simulink model "DAS"  (R2012b)
settings: Solver=FixedStepDiscrete  StartTime=0.0  StopTime=inf  FixedStep=0.1  RelTol=1e-3
PreLoadFcn:
  | if exist('tl_preloadfcn','file'), tl_preloadfcn(gcs,101); end
PostLoadFcn:
  | if exist('tl_postloadfcn','file'), tl_postloadfcn(gcs,101); end
InitFcn:
  | if exist('tlds_init','file'), tlds_init(gcs); end
StartFcn:
  | if exist('tlds_start','file'), tlds_start(gcs); end
StopFcn:
  | if exist('tlds_stop','file'), tlds_stop(gcs); end
undefined symbols (not defined in the file): A, B, C, Dd, DEMO_FAS_Accusti_Threshold_Time, DEMO_FAS_BrakeBooster_Threshold, DEMO_FAS_CC_DELTA, DEMO_FAS_CC_Lvl2_Round, DEMO_FAS_CC_Min_Value, DEMO_FAS_Distance_Treshold_Far, DEMO_FAS_Distance_Treshold_Med, DEMO_FAS_Distance_Treshold_Near, DEMO_FAS_Distronic, DEMO_FAS_Emerg_Brake_Force1, DEMO_FAS_Emerg_Brake_Force2, DEMO_FAS_Emerg_Brake_Time1, DEMO_FAS_Emerg_Brake_Time2, DEMO_FAS_EmergencyBrake, DEMO_FAS_FollowToStop, DEMO_FAS_Limiter, DEMO_FAS_Limiter_DELTA, DEMO_FAS_Neg_Max_ms, DEMO_FAS_Opti_Threshold_Time, DEMO_FAS_Repeater, DEMO_FAS_Repeater_Time, DEMO_FAS_Signdetection, DEMO_FAS_Tempomat
(part 1 of 11)
PreSaveFcn:
  | if exist('tl_presavefcn','file'), tl_presavefcn(gcs); end
settings Model: TL_MAIN_DATA={'date',735360.45236349537}  TLRevision=101  DS_PROJECTFILE=Oeffentlicher_Demonstrator_FAS.dd  BufferReuse=off  Creator=YVEDUHR  LastModifiedBy=alex
settings OptimizationCC: BlockReduction=off  OptimizeBlockIOStorage=off  BufferReuse=off  ExpressionFolding=off  LocalBlockOutputs=off
settings DebuggingCC: InheritedTsInSrcMsg=none

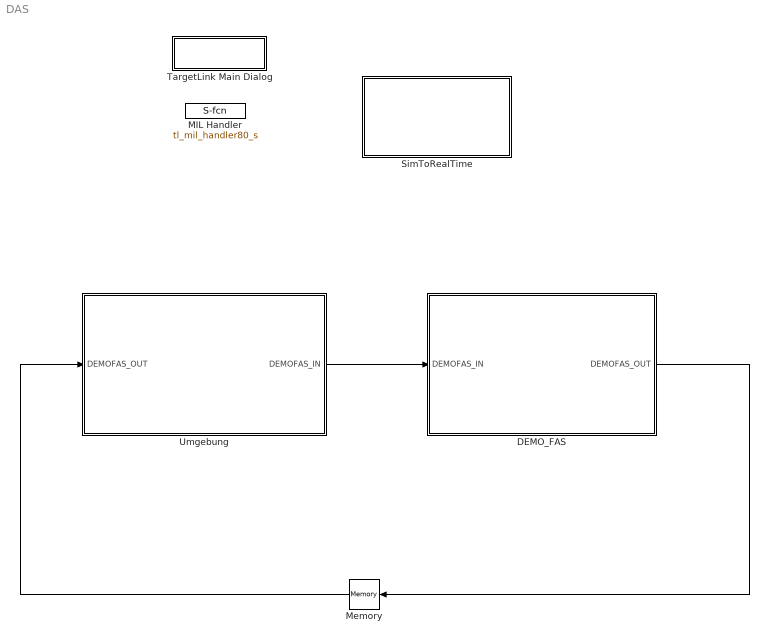
== system DAS ==
  DEMO_FAS : Subsystem
  MIL Handler : S-Function  FunctionName=tl_mil_handler80_s  EnableBusSupport=off  mask(TL_MilHandler){data={'date',730486}}
      mask help: TargetLink MIL Handler
      mask init:
      | fname = sprintf('tl_mil_handler%d_s', 10*get_param(0,'Version'));
      | set_param(gcbh,'FunctionName', fname, 'SFunctionModules','''''');
      settings: DeleteFcn=if exist('delete_tlblock','file')==2,delete_tlblock(gcbh);end  NameChangeFcn=if exist('rename_tlblock','file')==2,rename_tlblock(gcbh);end  OpenFcn=open_system(gcbh,'mask')
      mask Help: eval('if exist(''tl_online_help'',''file'') == 2, tl_online_help(''Topic'',get_param(gcbh,''MaskType'')),end')
      mask Display: disp('MIL Handler')
  Memory : Memory
  SimToRealTime : Subsystem
  TargetLink Main Dialog : Subsystem  mask(TL_MainDialog){data=[]}
      mask help: TargetLink Main Dialog block: In full-featured mode it provides the main graphical user interface to TargetLink.
      mask init:
      | if exist('tl_get_blockset_mode','file')==2
      |    if strcmp(tl_get_blockset_mode,'full-featured')
      |       set_param(gcbh,'BackgroundColor','green');
      |    else
      |       set_param(gcbh,'BackgroundColor','[0.6,0.6,0.6]');
      |    end
      | else
      |    set_param(gcbh,'BackgroundColor','[0.6,0.6,0.6]');
      | end
      settings: CopyFcn=if exist('tl_copyfcn') == 2, tl_copyfcn(gcbh); end
      settings: OpenFcn=|
      | if exist('tl_open_blockdlg','file')==2
      |     tl_open_blockdlg(gcbh);
      | else
      |     open_system(gcbh,'mask');
      | end
      mask Help: eval('if exist(''tl_online_help'',''file'') == 2, tl_online_help(''Topic'',get_param(gcbh,''MaskType'')),end')
      mask Display: disp('TargetLink')
  Umgebung : Subsystem
  wires:
  DEMO_FAS/1(DEMOFAS_OUT) -> Memory/1
  Memory/1 -> Umgebung/1(DEMOFAS_OUT)
  Umgebung/1(DEMOFAS_IN) -> DEMO_FAS/1(DEMOFAS_IN)

== system DAS/DEMO_FAS ==
  DEMOFAS_IN : Inport
  Bus Creator : BusCreator  Inputs=8
  Bus Selector : BusSelector  OutputSignals=ParkingBrake_b,BrakeForce_pedal_pc,Accelaration_pedal_pc,CruiseControl_b,Limiter_b,LeverUp_stat,LeverDown_stat,V_Vehicle_kmh,V_Sign_kmh,Sign_b,Distance_stat,V_Obj_rel_kmh,Distance_Object_m
  DEMO_FAS : Subsystem  Tag=TargetLink Simulation Frame  mask(TL_SimFrame){}
      settings: CopyFcn=if exist('tl_copyfcn','file'), tl_copyfcn(gcbh); end  NameChangeFcn=if exist('tl_framenamechangefcn','file'), tl_framenamechangefcn(gcbh); end
      settings: OpenFcn=|
      | if exist('open_tlsubsystem','file')
      |    open_tlsubsystem(gcbh);
      | else
      |    tlsubsystem = ...
      |       find_system(gcb, ...
      |       'LookUnderMasks','on', ...
      |       'FollowLinks','on', ...
      |       'Tag','MIL Subsystem');
      |    open_system(tlsubsystem);
      | end
      mask Display: disp('TargetLink\nModel-\nin-the-loop\nmode')
  DEMOFAS_OUT : Outport
  wires:
  Bus Creator/1 -> DEMOFAS_OUT/1
  DEMOFAS_IN/1 -> Bus Selector/1
  DEMO_FAS/3(_BrakeForce_pc) -> Bus Creator/3
  DEMO_FAS/6(_Limiter_active_b) -> Bus Creator/6
  DEMO_FAS/5(_LimiterSetValue_kmh) -> Bus Creator/5
  DEMO_FAS/4(_CCSetValue_kmh) -> Bus Creator/4
  DEMO_FAS/2(_Acceleration_pc) -> Bus Creator/2
  DEMO_FAS/1(_CC_active_b) -> Bus Creator/1
  Bus Selector/12 -> DEMO_FAS/12(_V_Obj_rel_kmh)  "<V_Obj_rel_kmh>"
  Bus Selector/13 -> DEMO_FAS/13(_Distance_Object_m)  "<Distance_Object_m>"
  Bus Selector/10 -> DEMO_FAS/10(_Sign_b)  "<Sign_b>"
  Bus Selector/9 -> DEMO_FAS/9(_V_Sign_kmh)  "<V_Sign_kmh>"
  Bus Selector/3 -> DEMO_FAS/3(_Accelaration_pedal_pc)  "<Accelaration_pedal_pc>"
  Bus Selector/4 -> DEMO_FAS/4(_CruiseControl_b)  "<CruiseControl_b>"
  Bus Selector/5 -> DEMO_FAS/5(_Limiter_b)  "<Limiter_b>"
  Bus Selector/2 -> DEMO_FAS/2(_BrakeForce_pedal_pc)  "<BrakeForce_pedal_pc>"
  Bus Selector/7 -> DEMO_FAS/7(_LeverDown_stat)  "<LeverDown_stat>"
  Bus Selector/6 -> DEMO_FAS/6(_LeverUp_stat)  "<LeverUp_stat>"
  Bus Selector/1 -> DEMO_FAS/1(_ParkingBrake_b)  "<ParkingBrake_b>"
  Bus Selector/8 -> DEMO_FAS/8(_V_Vehicle_kmh)  "<V_Vehicle_kmh>"
  Bus Selector/11 -> DEMO_FAS/11(_Distance_stat)  "<Distance_stat>"
  DEMO_FAS/7(_Opti_warn_b) -> Bus Creator/7
  DEMO_FAS/8(_Acusti_warn_b) -> Bus Creator/8

== system DAS/SimToRealTime ==
  Constant : Constant  Value=0
  Constant1 : Constant
  Terminator{,1..5} (6 alike) : Terminator
  VAPS_TimeConfiguration : Subsystem  mask(SL_ACT_SG_VAPS_TimeConfiguration_V100){ts=-1}
      mask prompts: ts "Sample Time"
      mask help:
      | This Blocks syncs if possible the simulation with the real time clock
      | with special features for VAPS
      |
      | This Block has the following Inputs- and Output Signals
      |
      | Input:
      | - TimeConfig: Value [from -10 to 10] to increase or decrease the simulation speed
      |
      | Example:
      |
      | Value:            -10 | -9 | -8 | -7 | -6 | -5 | -4 | -3 | -2 | -1| 0 | 1 | 2 | 3 | 4 | 5 | 6 | 7 | 8 | 9 | 10
      | -----------------------------------------------------------------------------------------------------------------------------------
      | TimeFactor:    0.1|0.9|0.8|0.7|0.6|0.5|0.4|0.3|0.2|0.1| 1 | 1 | 2 | 3 | 4 | 5 | 6 | 7 | 8 | 9 | 10
      |
      | TimeConfig=10 --> :Run 10x faster than Real Time
      | TimeConfig= -5 --> :Run 0.5x as fast than Real Time
      |
      |   -  -1< TimeConfig < 1  	: Run at Real Time
      |    - TimeConfig >1	: Run faster than RealTime
      |    - TimeConfig <-1	: Run slower than RealTime
      |
      | - MaxSpeed:
      |    - MaxSpeed =1	: Run at Real Time with TimeFactor
      |    - MaxSpeed =2	: Run as fast as possible
      |
      | Output:
      | - Factor_SimTime: TimeFactor for the execution SampleTime
      | - TimeConfig_Consumer: TimeConfig for VAPS TimeFactor_Consumer
      | - TimeConfig_Producer: TimeConfig for writing into the TimeConfig_Producer channel
      | - TsSim: SampleTime of the Simulation
      | - TsRTime:Realtime execution SampleTime
      | - TsRTimeEffective: Effective Realtime execution Time
      |
      | Parameter:
      | - Sample Time: execution SampleTime
  wires:
  Constant/1 -> VAPS_TimeConfiguration/1(TimeConfig)
  Constant1/1 -> VAPS_TimeConfiguration/2(MaxSpeed)
  VAPS_TimeConfiguration/1(Factor_SimTime) -> Terminator/1
  VAPS_TimeConfiguration/2(TimeConfig_Consumer) -> Terminator1/1
  VAPS_TimeConfiguration/6(TsRTimeEff) -> Terminator5/1
  VAPS_TimeConfiguration/5(TsRTime) -> Terminator4/1
  VAPS_TimeConfiguration/4(TsSim) -> Terminator3/1
  VAPS_TimeConfiguration/3(TimeConfig_Producer) -> Terminator2/1

== system DAS/TargetLink Main Dialog ==
  dSPACE logo : Subsystem
      mask Display: image(ds_get_icon('dspace_logo_bg_white_l'))

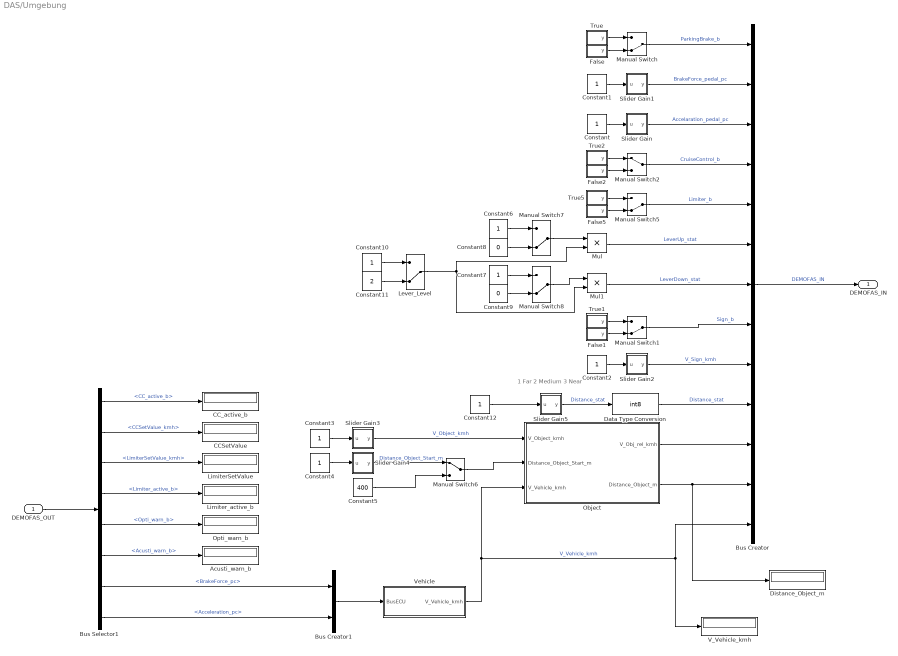
== system DAS/Umgebung ==
  note: 1 Far
      | 2 Medium
      | 3 Near
  DEMOFAS_OUT : Inport
  Acusti_warn_b : Display
  Bus Selector1 : BusSelector  OutputSignals=CC_active_b,CCSetValue_kmh,LimiterSetValue_kmh,Limiter_active_b,Opti_warn_b,Acusti_warn_b,BrakeForce_pc,Acceleration_pc
  Bus Creator : BusCreator  Inputs=13
  Bus Creator1 : BusCreator  Inputs=2
  CCSetValue : Display
  CC_active_b : Display
  Constant{,1..4,6..7,10,12} (9 alike) : Constant
  Constant11 : Constant  Value=2
  Constant5 : Constant  Value=400
  Constant8 : Constant  Value=0
  Constant9 : Constant  Value=0
  Data Type Conversion : DataTypeConversion  OutMin=1  OutMax=3  OutDataTypeStr=int8
  Distance_Object_m : Display
  False : Subsystem  mask(ACT_SG_V200_False){}
      mask help: False
      mask Display: disp('False');
  False1 : Subsystem  mask(ACT_SG_V200_False){}
      mask help: False
      mask Display: disp('False');
  False2 : Subsystem  mask(ACT_SG_V200_False){}
      mask help: False
      mask Display: disp('False');
  False5 : Subsystem  mask(ACT_SG_V200_False){}
      mask help: False
      mask Display: disp('False');
  Lever_Level : ManualSwitch  CurrentSetting=0
  LimiterSetValue : Display
  Limiter_active_b : Display
  Manual Switch{,1,5,7..8} (5 alike) : ManualSwitch  CurrentSetting=0
  Manual Switch2 : ManualSwitch
  Manual Switch6 : ManualSwitch
  Mul : Product  SaturateOnIntegerOverflow=on  InputSameDT=on  OutDataTypeStr=Inherit: Same as first input
  Mul1 : Product  SaturateOnIntegerOverflow=on  InputSameDT=on  OutDataTypeStr=Inherit: Same as first input
  Object : Subsystem
  Opti_warn_b : Display
  Slider Gain : Subsystem  LoadFcn=slideg Load  StartFcn=slideg StartFcn  StopFcn=slideg StopFcn  mask(Slider Gain){low=0, gain=50, high=100}
      mask prompts: low "Simulink:masks:Low_MP"; gain "Simulink:masks:Gain_MP"; high "Simulink:masks:High_MP"
      settings: CopyFcn=slideg Copy  DeleteFcn=slideg DeleteBlock  NameChangeFcn=slideg NameChange  OpenFcn=slideg Open  CloseFcn=slideg Close  ParentCloseFcn=slideg ParentClose
      mask Display: disp(gain)
  Slider Gain1 : Subsystem  LoadFcn=slideg Load  StartFcn=slideg StartFcn  StopFcn=slideg StopFcn  mask(Slider Gain){low=0, gain=0, high=100}
      mask prompts: low "Simulink:masks:Low_MP"; gain "Simulink:masks:Gain_MP"; high "Simulink:masks:High_MP"
      settings: CopyFcn=slideg Copy  DeleteFcn=slideg DeleteBlock  NameChangeFcn=slideg NameChange  OpenFcn=slideg Open  CloseFcn=slideg Close  ParentCloseFcn=slideg ParentClose
      mask Display: disp(gain)
  Slider Gain2 : Subsystem  LoadFcn=slideg Load  StartFcn=slideg StartFcn  StopFcn=slideg StopFcn  mask(Slider Gain){low=0, gain=50, high=100}
      mask prompts: low "Simulink:masks:Low_MP"; gain "Simulink:masks:Gain_MP"; high "Simulink:masks:High_MP"
      settings: CopyFcn=slideg Copy  DeleteFcn=slideg DeleteBlock  NameChangeFcn=slideg NameChange  OpenFcn=slideg Open  CloseFcn=slideg Close  ParentCloseFcn=slideg ParentClose
      mask Display: disp(gain)
  Slider Gain3 : Subsystem  LoadFcn=slideg Load  StartFcn=slideg StartFcn  StopFcn=slideg StopFcn  mask(Slider Gain){low=0, gain=30, high=250}
      mask prompts: low "Simulink:masks:Low_MP"; gain "Simulink:masks:Gain_MP"; high "Simulink:masks:High_MP"
      settings: CopyFcn=slideg Copy  DeleteFcn=slideg DeleteBlock  NameChangeFcn=slideg NameChange  OpenFcn=slideg Open  CloseFcn=slideg Close  ParentCloseFcn=slideg ParentClose
      mask Display: disp(gain)
  Slider Gain4 : Subsystem  LoadFcn=slideg Load  StartFcn=slideg StartFcn  StopFcn=slideg StopFcn  mask(Slider Gain){low=0, gain=50, high=300}
      mask prompts: low "Simulink:masks:Low_MP"; gain "Simulink:masks:Gain_MP"; high "Simulink:masks:High_MP"
      settings: CopyFcn=slideg Copy  DeleteFcn=slideg DeleteBlock  NameChangeFcn=slideg NameChange  OpenFcn=slideg Open  CloseFcn=slideg Close  ParentCloseFcn=slideg ParentClose
      mask Display: disp(gain)
  Slider Gain5 : Subsystem  LoadFcn=slideg Load  StartFcn=slideg StartFcn  StopFcn=slideg StopFcn  mask(Slider Gain){low=1, gain=2.36, high=3}
      mask prompts: low "Simulink:masks:Low_MP"; gain "Simulink:masks:Gain_MP"; high "Simulink:masks:High_MP"
      settings: CopyFcn=slideg Copy  DeleteFcn=slideg DeleteBlock  NameChangeFcn=slideg NameChange  OpenFcn=slideg Open  CloseFcn=slideg Close  ParentCloseFcn=slideg ParentClose
      mask Display: disp(gain)
  True : Subsystem  mask(ACT_SG_V200_True){}
      mask help: True
      mask Display: disp('True')
  True1 : Subsystem  mask(ACT_SG_V200_True){}
      mask help: True
      mask Display: disp('True')
  True2 : Subsystem  mask(ACT_SG_V200_True){}
      mask help: True
      mask Display: disp('True')
  True5 : Subsystem  mask(ACT_SG_V200_True){}
      mask help: True
      mask Display: disp('True')
  V_Vehicle_kmh : Display
  Vehicle : Subsystem
  DEMOFAS_IN : Outport
  wires:
  Bus Creator/1 -> DEMOFAS_IN/1  "DEMOFAS_IN"
  True/1(y) -> Manual Switch/1
  False/1(y) -> Manual Switch/2
  Manual Switch/1 -> Bus Creator/1  "ParkingBrake_b"
  Slider Gain1/1(y) -> Bus Creator/2  "BrakeForce_pedal_pc"
  True2/1(y) -> Manual Switch2/1
  False2/1(y) -> Manual Switch2/2
  Manual Switch2/1 -> Bus Creator/4  "CruiseControl_b"
  True5/1(y) -> Manual Switch5/1
  False5/1(y) -> Manual Switch5/2
  Manual Switch5/1 -> Bus Creator/5  "Limiter_b"
  Vehicle/1(V_Vehicle_kmh) -> Object/3(V_Vehicle_kmh), Bus Creator/13, V_Vehicle_kmh/1  "V_Vehicle_kmh"
  Bus Creator1/1 -> Vehicle/1(BusECU)
  DEMOFAS_OUT/1 -> Bus Selector1/1
  Bus Selector1/8 -> Bus Creator1/2  "<Acceleration_pc>"
  Constant/1 -> Slider Gain/1(u)
  Slider Gain/1(y) -> Bus Creator/3  "Accelaration_pedal_pc"
  Constant1/1 -> Slider Gain1/1(u)
  Bus Selector1/1 -> CC_active_b/1  "<CC_active_b>"
  Bus Selector1/2 -> CCSetValue/1  "<CCSetValue_kmh>"
  Bus Selector1/3 -> LimiterSetValue/1  "<LimiterSetValue_kmh>"
  Bus Selector1/4 -> Limiter_active_b/1  "<Limiter_active_b>"
  Bus Selector1/7 -> Bus Creator1/1  "<BrakeForce_pc>"
  True1/1(y) -> Manual Switch1/1
  False1/1(y) -> Manual Switch1/2
  Manual Switch1/1 -> Bus Creator/8  "Sign_b"
  Constant2/1 -> Slider Gain2/1(u)
  Slider Gain2/1(y) -> Bus Creator/9  "V_Sign_kmh"
  Constant3/1 -> Slider Gain3/1(u)
  Slider Gain3/1(y) -> Object/1(V_Object_kmh)  "V_Object_kmh"
  Constant4/1 -> Slider Gain4/1(u)
  Slider Gain4/1(y) -> Manual Switch6/1  "Distance_Object_Start_m"
  Constant5/1 -> Manual Switch6/2
  Manual Switch6/1 -> Object/2(Distance_Object_Start_m)
  Object/1(V_Obj_rel_kmh) -> Bus Creator/11
  Object/2(Distance_Object_m) -> Distance_Object_m/1, Bus Creator/12
  Constant6/1 -> Manual Switch7/1
  Constant7/1 -> Manual Switch8/1
  Constant8/1 -> Manual Switch7/2
  Constant9/1 -> Manual Switch8/2
  Mul/1 -> Bus Creator/6  "LeverUp_stat"
  Manual Switch7/1 -> Mul/1
  Constant10/1 -> Lever_Level/1
  Constant11/1 -> Lever_Level/2
  Lever_Level/1 -> Mul/2, Mul1/2
  Mul1/1 -> Bus Creator/7  "LeverDown_stat"
  Manual Switch8/1 -> Mul1/1
  Slider Gain5/1(y) -> Data Type Conversion/1  "Distance_stat"
  Constant12/1 -> Slider Gain5/1(u)
  Data Type Conversion/1 -> Bus Creator/10  "Distance_stat"
  Bus Selector1/5 -> Opti_warn_b/1  "<Opti_warn_b>"
  Bus Selector1/6 -> Acusti_warn_b/1  "<Acusti_warn_b>"

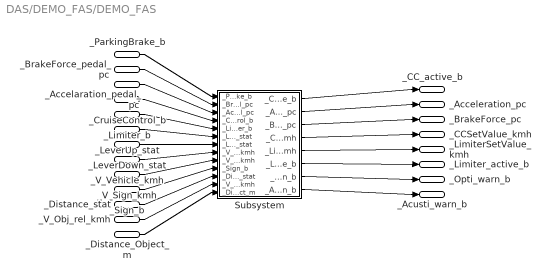
== system DAS/DEMO_FAS/DEMO_FAS ==
  _ParkingBrake_b : Inport
  _BrakeForce_pedal_pc : Inport  Port=2
  _Accelaration_pedal_pc : Inport  Port=3
  _CruiseControl_b : Inport  Port=4
  _Limiter_b : Inport  Port=5
  _LeverUp_stat : Inport  Port=6
  _LeverDown_stat : Inport  Port=7
  _V_Vehicle_kmh : Inport  Port=8
  _V_Sign_kmh : Inport  Port=9
  _Sign_b : Inport  Port=10
  _Distance_stat : Inport  Port=11
  _V_Obj_rel_kmh : Inport  Port=12
  _Distance_Object_m : Inport  Port=13
  Subsystem : Subsystem  Tag=struct('sfcnName','DEMO_FAS_sf','subFunction','','srcSubsystem','')  mask(TL_Enable){}
      settings: OpenFcn=warndlg(get_param(gcb,'MaskHelp'),'Serious Warning');
      mask Help: This subsystem keeps the TargetLink subsystem (subsystem with TargetLink blocks for production code generation), and is needed for the TargetLink simulation frame to work properly. DO NOT DELETE OR MODIFY IT!
  _CC_active_b : Outport
  _Acceleration_pc : Outport  Port=2
  _BrakeForce_pc : Outport  Port=3
  _CCSetValue_kmh : Outport  Port=4
  _LimiterSetValue_kmh : Outport  Port=5
  _Limiter_active_b : Outport  Port=6
  _Opti_warn_b : Outport  Port=7
  _Acusti_warn_b : Outport  Port=8
  wires:
  _ParkingBrake_b/1 -> Subsystem/1(_ParkingBrake_b)
  _BrakeForce_pedal_pc/1 -> Subsystem/2(_BrakeForce_pedal_pc)
  _Accelaration_pedal_pc/1 -> Subsystem/3(_Accelaration_pedal_pc)
  _CruiseControl_b/1 -> Subsystem/4(_CruiseControl_b)
  _Limiter_b/1 -> Subsystem/5(_Limiter_b)
  _LeverUp_stat/1 -> Subsystem/6(_LeverUp_stat)
  _LeverDown_stat/1 -> Subsystem/7(_LeverDown_stat)
  _V_Vehicle_kmh/1 -> Subsystem/8(_V_Vehicle_kmh)
  _V_Sign_kmh/1 -> Subsystem/9(_V_Sign_kmh)
  _Sign_b/1 -> Subsystem/10(_Sign_b)
  _Distance_stat/1 -> Subsystem/11(_Distance_stat)
  _V_Obj_rel_kmh/1 -> Subsystem/12(_V_Obj_rel_kmh)
  _Distance_Object_m/1 -> Subsystem/13(_Distance_Object_m)
  Subsystem/1(_CC_active_b) -> _CC_active_b/1
  Subsystem/2(_Acceleration_pc) -> _Acceleration_pc/1
  Subsystem/3(_BrakeForce_pc) -> _BrakeForce_pc/1
  Subsystem/4(_CCSetValue_kmh) -> _CCSetValue_kmh/1
  Subsystem/5(_LimiterSetValue_kmh) -> _LimiterSetValue_kmh/1
  Subsystem/6(_Limiter_active_b) -> _Limiter_active_b/1
  Subsystem/7(_Opti_warn_b) -> _Opti_warn_b/1
  Subsystem/8(_Acusti_warn_b) -> _Acusti_warn_b/1

== system DAS/SimToRealTime/VAPS_TimeConfiguration ==
  TimeConfig : Inport
  MaxSpeed : Inport  Port=2
  Constant1 : Constant  Value=0
  Constant10 : Constant  Value=2
  Constant4 : Constant  Value=0
  RealTimeTimerAdapter : Subsystem
  RealTimeTimerAdapter_Value : Subsystem
  RelOp4 : RelationalOperator  Operator===  InputSameDT=on
  Switch1 : Switch  Threshold=1  SaturateOnIntegerOverflow=on  InputSameDT=on
  Switch2 : Switch  Threshold=1  SaturateOnIntegerOverflow=on  InputSameDT=on
  SysInit1 : Subsystem  mask(ACT_SG_V200_SysInit){dT=ts, YName=}
      mask prompts: dT "Sample Time"; YName "Y OutName"
      mask help: An inital pulse is generated for for the first block evaluation.
      mask init:
      | sl_act_sg_init_blk;
      mask Help:
      | <P><B>Function:</B></P>
      | <P>The block provides an initial pulse at the output on the first
      | evaluation of the block.<BR> This function can be used for system startup functions to
      | get defined states in the system.</P>
      | 
      | <P><B>In-/Outputs:</B></P>
      | <P><U>Output</U></P>
      | <P>The output shows TRUE at the first cycle, else it shows FALSE.</P>
      mask Display: disp('SysInit');
  VAPSRealTimeTimer : Subsystem  mask(SL_ACT_SG_VAPSRealTimeTimer_V100){}
      mask help:
      | This Blocks syncs if possible the simulation with the real time clock.
      |
      | This Block has the following Inputs- and Output Signals
      |
      | Input:
      | - TimeFactor: Factor to increase or decrease the simulation speed
      |    - TimeFactor =1  	: Run at Real Time
      |    - TimeFactor >1	: Run TimeFactor faster than RealTime
      |    - TimeFactor <1	: Run TimeFactor slower than RealTime
      |    - TimeFactor =0	: Run as fast as possible
      |
      | Output:
      | - TsSim: SampleTime of the Simulation
      | - TsRTime:Realtime execution SampleTime
      | - TsRTimeEffective: Effective Realtime execution Time
  Factor_SimTime : Outport
  TimeConfig_Consumer : Outport  Port=2
  TimeConfig_Producer : Outport  Port=3
  TsSim : Outport  Port=4
  TsRTime : Outport  Port=5
  TsRTimeEff : Outport  Port=6
  wires:
  Switch2/1 -> RealTimeTimerAdapter/1(In1), RealTimeTimerAdapter_Value/1(In1)
  Constant4/1 -> Switch2/1
  SysInit1/1(y) -> Switch2/2
  TimeConfig/1 -> Switch2/3
  RealTimeTimerAdapter/1(Out1) -> Factor_SimTime/1, Switch1/3
  RealTimeTimerAdapter_Value/1(Out1) -> TimeConfig_Consumer/1, TimeConfig_Producer/1
  VAPSRealTimeTimer/1(TsSim) -> TsSim/1
  VAPSRealTimeTimer/2(TsRTime) -> TsRTime/1
  VAPSRealTimeTimer/3(TsRTimeEffective) -> TsRTimeEff/1
  Constant10/1 -> RelOp4/2
  Switch1/1 -> VAPSRealTimeTimer/1(TimeFactor)
  RelOp4/1 -> Switch1/2
  MaxSpeed/1 -> RelOp4/1
  Constant1/1 -> Switch1/1

== system DAS/TargetLink Main Dialog/dSPACE logo ==

== system DAS/Umgebung/False ==
  Zero : Constant  Value=0
  y : Outport
  wires:
  Zero/1 -> y/1

== system DAS/Umgebung/False1 ==
  Zero : Constant  Value=0
  y : Outport
  wires:
  Zero/1 -> y/1

== system DAS/Umgebung/False2 ==
  Zero : Constant  Value=0
  y : Outport
  wires:
  Zero/1 -> y/1

== system DAS/Umgebung/False5 ==
  Zero : Constant  Value=0
  y : Outport
  wires:
  Zero/1 -> y/1

== system DAS/Umgebung/Object ==
  V_Object_kmh : Inport
  Distance_Object_Start_m : Inport  Port=2
  V_Vehicle_kmh : Inport  Port=3
  Accumulator_REL : Subsystem  mask(MSR_V200_AccumulatorResetEnabledLimited){dT=-1, YName=, b_maxName=, b_minName=}
      mask prompts: dT "Sample Time"; YName "Y OutName"; b_maxName "b_max OutName"; b_minName "b_min OutName"
      mask help:
      | 'y' is the sum of all sampled input values 'u', limited to 'MN' and 'MX'.
      | 'E' on FALSE stops the integration.
      | 'R' on TRUE loads initial value 'IV'.
      | 'y' on limit is indicated by 'b_max' and 'b_min' flags.
      mask init:
      | sl_act_sg_init_blk;
      mask Help:
      | <HTML>
      | <HEAD>
      | <META HTTP-EQUIV="Content-Type" CONTENT="text/html; charset=iso-8859-1">
      | <TITLE>Help</TITLE>
      | </HEAD>
      | <BODY>
      | 
      | <B><FONT FACE="Arial"><P>Function:</P>
      | </B><P>The block works as a totalizer of the input signal
      |  <FONT FACE="Courier New">u</FONT>.</P>
      | 
      | <B><P>In-/Outputs:</P>
      | </B>
      | <P><U>Enable</U></P>
      | <P> If the enable input <FONT FACE="Courier New">E</FONT> is '0' the
      | 	 calculation is stopped and the output
      | 	 <FONT FACE="Courier New">y</FONT> shows the last evaluated value.</P>
      | 
      | <P><U>Input</U></P>
      | <P>The block input <FONT FACE="Courier New">u</FONT> must be connected
      | 	 to the input signal.</P>
      | 
      | <U><P>Reset / Initial Value</P>
      | </U><P>If the reset input <FONT FACE="Courier New">R</FONT>
      | <FONT FACE="Arial"> gets a '1' signal the block will output the initial value
      |  <FONT FACE="Courier New">IV</FONT>.</P>
      | 
      | <U><P>Limit Values</P>
      | </U><P>The inputs <FONT FACE="Courier New">MN</FONT> and
      |  <FONT FACE="Courier New">MX</FONT> specify the signal value limits for
      |   <FONT FACE="Courier New">y</FONT>.</P>
      | 
      | <U><P>Output</P>
      | </U><P>The output <FONT FACE="Courier New">y</FONT> shows the totalized
      |  input signal, limited to <FONT FACE="Courier New">MN</FONT> and
      |   <FONT FACE="Courier New">MX</FONT>.<BR>
      | 	 <FONT FACE="Courier New">b_min</FONT>
      | 	 and <FONT FACE="Courier New">b_max</FONT> indicate that the totalized
      | 	  signal has reached the minimum resp. the maximum.</P>
      | </FONT></BODY>
      | </HTML>
      mask Display: image(imread('Accumulator.tif','tif'),[0.25,0.2,0.3,0.6])
  Add : Sum  Inputs=+-
  Constant : Constant  Value=300
  Constant1 : Constant  Value=1000
  Constant2 : Constant  Value=0
  Gain : Gain  Gain=-1/3.6
  Logical Operator : Logic  Operator=NOT  AllPortsSameDT=off  OutDataTypeStr=boolean
  RelOp : RelationalOperator  Operator=>  InputSameDT=on
  Terminator : Terminator
  Terminator1 : Terminator
  V_Obj_rel_kmh : Outport
  Distance_Object_m : Outport  Port=2
  wires:
  V_Object_kmh/1 -> Add/2
  V_Vehicle_kmh/1 -> Add/1
  Add/1 -> Gain/1, V_Obj_rel_kmh/1  "V_Obj_rel_kmh"
  Gain/1 -> Accumulator_REL/3(u)
  Constant/1 -> RelOp/2
  Distance_Object_Start_m/1 -> RelOp/1, Accumulator_REL/6(IV)
  RelOp/1 -> Logical Operator/1, Accumulator_REL/5(R)
  Constant1/1 -> Accumulator_REL/1(MX)
  Constant2/1 -> Accumulator_REL/2(MN)
  Accumulator_REL/1(y) -> Distance_Object_m/1  "Distance_Object_m"
  Logical Operator/1 -> Accumulator_REL/4(E)
  Accumulator_REL/2(b_max) -> Terminator/1
  Accumulator_REL/3(b_min) -> Terminator1/1

== system DAS/Umgebung/Slider Gain ==
  u : Inport
  Slider Gain : Gain  Gain=gain  SaturateOnIntegerOverflow=on  OutDataTypeStr=Inherit: Same as input  ParamDataTypeStr=Inherit: Same as input
  y : Outport
  wires:
  u/1 -> Slider Gain/1
  Slider Gain/1 -> y/1

== system DAS/Umgebung/Slider Gain1 ==
  u : Inport
  Slider Gain : Gain  Gain=gain  SaturateOnIntegerOverflow=on  OutDataTypeStr=Inherit: Same as input  ParamDataTypeStr=Inherit: Same as input
  y : Outport
  wires:
  u/1 -> Slider Gain/1
  Slider Gain/1 -> y/1

== system DAS/Umgebung/Slider Gain2 ==
  u : Inport
  Slider Gain : Gain  Gain=gain  SaturateOnIntegerOverflow=on  OutDataTypeStr=Inherit: Same as input  ParamDataTypeStr=Inherit: Same as input
  y : Outport
  wires:
  u/1 -> Slider Gain/1
  Slider Gain/1 -> y/1

== system DAS/Umgebung/Slider Gain3 ==
  u : Inport
  Slider Gain : Gain  Gain=gain  SaturateOnIntegerOverflow=on  OutDataTypeStr=Inherit: Same as input  ParamDataTypeStr=Inherit: Same as input
  y : Outport
  wires:
  u/1 -> Slider Gain/1
  Slider Gain/1 -> y/1

== system DAS/Umgebung/Slider Gain4 ==
  u : Inport
  Slider Gain : Gain  Gain=gain  SaturateOnIntegerOverflow=on  OutDataTypeStr=Inherit: Same as input  ParamDataTypeStr=Inherit: Same as input
  y : Outport
  wires:
  u/1 -> Slider Gain/1
  Slider Gain/1 -> y/1

== system DAS/Umgebung/Slider Gain5 ==
  u : Inport
  Slider Gain : Gain  Gain=gain  SaturateOnIntegerOverflow=on  OutDataTypeStr=Inherit: Same as input  ParamDataTypeStr=Inherit: Same as input
  y : Outport
  wires:
  u/1 -> Slider Gain/1
  Slider Gain/1 -> y/1

== system DAS/Umgebung/True ==
  One : Constant
  y : Outport
  wires:
  One/1 -> y/1

== system DAS/Umgebung/True1 ==
  One : Constant
  y : Outport
  wires:
  One/1 -> y/1

== system DAS/Umgebung/True2 ==
  One : Constant
  y : Outport
  wires:
  One/1 -> y/1

== system DAS/Umgebung/True5 ==
  One : Constant
  y : Outport
  wires:
  One/1 -> y/1

== system DAS/Umgebung/Vehicle ==
  BusECU : Inport
  Bus Selector : BusSelector  OutputSignals=BrakeForce_pc,Acceleration_pc
  Constant : Constant  Value=0
  Constant1 : Constant  Value=0
  Discrete Transfer Fcn (with initial states) : Subsystem  mask(Discrete Transfer Function with Initial States){N=[0.009975], D=[1  -0.997], X0=[1], TS=.1}
      mask prompts: N "SimulinkBlocks:simulink_extras:Numerator_MP"; D "SimulinkBlocks:simulink_extras:Denominator_MP"; X0 "SimulinkBlocks:simulink_extras:InitialConditions_MP"; TS "SimulinkBlocks:simulink_extras:SampleTime_MP"
      mask help: SimulinkBlocks:simulink_extras:DiscreteTransferFunctionWithInitialStates_MD
      mask init:
      | [A,B,C,Dd]=tf2ss(N,D);if (isempty(X0));[m,n]=size(A);X0=zeros(1,m); end;
      mask Help: Specify the initial states for the transfer function.  The state ordering is determined by the m-file tf2ss.  There is no unique mapping of the states in a transfer function to states in a state-space representation.  However, tf2ss will consistently use the same mapping for a given transfer function.
      mask Display: dpoly(N,D,'z')
  Gain : Gain  Gain=-2
  Relational Operator : RelationalOperator  Operator=<  OutDataTypeStr=boolean
  Saturation : Saturate  UpperLimit=250  LowerLimit=0
  Sum1 : Sum  Inputs=+--  SaturateOnIntegerOverflow=on  InputSameDT=on  OutDataTypeStr=Inherit: Same as first input
  Switch : Switch  Criteria=u2 > Threshold
  Switch1 : Switch  Threshold=1
  Uniform Random Number : UniformRandomNumber  Minimum=0  SampleTime=0.1
  Unit Delay : UnitDelay  SampleTime=-1
  Widerstand : Lookup  InputValues=[0 100 175 250]  Table=[0 8 18 33]  OutMax=[100]
  V_Vehicle_kmh : Outport
  wires:
  Saturation/1 -> Unit Delay/1, V_Vehicle_kmh/1  "V_Vehicle_kmh"
  Gain/1 -> Switch/1
  Switch/1 -> Discrete Transfer Fcn (with initial states)/1(In1)
  BusECU/1 -> Bus Selector/1
  Bus Selector/2 -> Switch/3  "<Acceleration_pc>"
  Sum1/1 -> Saturation/1
  Discrete Transfer Fcn (with initial states)/1(Out1) -> Sum1/1  "V_Vehicle_kmh"
  Widerstand/1 -> Sum1/2
  Unit Delay/1 -> Relational Operator/2, Widerstand/1
  Uniform Random Number/1 -> Sum1/3
  Constant/1 -> Relational Operator/1
  Relational Operator/1 -> Switch1/2
  Bus Selector/1 -> Switch1/1  "<BrakeForce_pc>"
  Switch1/1 -> Switch/2, Gain/1
  Constant1/1 -> Switch1/3

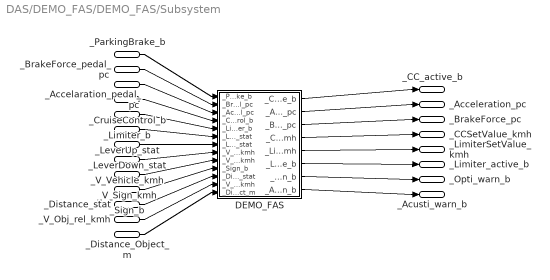
== system DAS/DEMO_FAS/DEMO_FAS/Subsystem ==
  _ParkingBrake_b : Inport
  _BrakeForce_pedal_pc : Inport  Port=2
  _Accelaration_pedal_pc : Inport  Port=3
  _CruiseControl_b : Inport  Port=4
  _Limiter_b : Inport  Port=5
  _LeverUp_stat : Inport  Port=6
  _LeverDown_stat : Inport  Port=7
  _V_Vehicle_kmh : Inport  Port=8
  _V_Sign_kmh : Inport  Port=9
  _Sign_b : Inport  Port=10
  _Distance_stat : Inport  Port=11
  _V_Obj_rel_kmh : Inport  Port=12
  _Distance_Object_m : Inport  Port=13
  DEMO_FAS : Subsystem  Tag=MIL Subsystem  Description=a  mask(MIL Subsystem){}
      settings: CopyFcn=if exist('tl_copyfcn','file'), tl_copyfcn(gcbh); end  NameChangeFcn=if exist('tl_namechangefcn','file'), tl_namechangefcn(gcbh); end  DestroyFcn=if exist('update_tl_main_dlg','file'), update_tl_main_dlg('TL_subs_display'); end
  _CC_active_b : Outport
  _Acceleration_pc : Outport  Port=2
  _BrakeForce_pc : Outport  Port=3
  _CCSetValue_kmh : Outport  Port=4
  _LimiterSetValue_kmh : Outport  Port=5
  _Limiter_active_b : Outport  Port=6
  _Opti_warn_b : Outport  Port=7
  _Acusti_warn_b : Outport  Port=8
  wires:
  _ParkingBrake_b/1 -> DEMO_FAS/1(_ParkingBrake_b)
  _BrakeForce_pedal_pc/1 -> DEMO_FAS/2(_BrakeForce_pedal_pc)
  _Accelaration_pedal_pc/1 -> DEMO_FAS/3(_Accelaration_pedal_pc)
  _CruiseControl_b/1 -> DEMO_FAS/4(_CruiseControl_b)
  _Limiter_b/1 -> DEMO_FAS/5(_Limiter_b)
  _LeverUp_stat/1 -> DEMO_FAS/6(_LeverUp_stat)
  _LeverDown_stat/1 -> DEMO_FAS/7(_LeverDown_stat)
  _V_Vehicle_kmh/1 -> DEMO_FAS/8(_V_Vehicle_kmh)
  _V_Sign_kmh/1 -> DEMO_FAS/9(_V_Sign_kmh)
  _Sign_b/1 -> DEMO_FAS/10(_Sign_b)
  _Distance_stat/1 -> DEMO_FAS/11(_Distance_stat)
  _V_Obj_rel_kmh/1 -> DEMO_FAS/12(_V_Obj_rel_kmh)
  _Distance_Object_m/1 -> DEMO_FAS/13(_Distance_Object_m)
  DEMO_FAS/1(_CC_active_b) -> _CC_active_b/1
  DEMO_FAS/2(_Acceleration_pc) -> _Acceleration_pc/1
  DEMO_FAS/3(_BrakeForce_pc) -> _BrakeForce_pc/1
  DEMO_FAS/4(_CCSetValue_kmh) -> _CCSetValue_kmh/1
  DEMO_FAS/5(_LimiterSetValue_kmh) -> _LimiterSetValue_kmh/1
  DEMO_FAS/6(_Limiter_active_b) -> _Limiter_active_b/1
  DEMO_FAS/7(_Opti_warn_b) -> _Opti_warn_b/1
  DEMO_FAS/8(_Acusti_warn_b) -> _Acusti_warn_b/1

== system DAS/SimToRealTime/VAPS_TimeConfiguration/RealTimeTimerAdapter ==
  In1 : Inport
  Constant1 : Constant  Value=-10
  Constant10 : Constant
  Constant11 : Constant
  Constant12 : Constant  Value=-1
  Constant13 : Constant
  Constant15 : Constant  Value=1.1
  Div1 : Product  Inputs=*/  SaturateOnIntegerOverflow=on  InputSameDT=on  OutDataTypeStr=Inherit: Same as first input
  LogOp1 : Logic
  RelOp2 : RelationalOperator  Operator=>  InputSameDT=on
  RelOp3 : RelationalOperator  Operator=<=  InputSameDT=on
  RelOp4 : RelationalOperator  InputSameDT=on
  Sum : Sum  Inputs=+-  SaturateOnIntegerOverflow=on  InputSameDT=on  OutDataTypeStr=Inherit: Same as first input
  Switch2 : Switch  Threshold=1  SaturateOnIntegerOverflow=on  InputSameDT=on
  Switch3 : Switch  Threshold=1  SaturateOnIntegerOverflow=on  InputSameDT=on
  Out1 : Outport
  wires:
  Div1/1 -> Sum/2
  Constant15/1 -> Sum/1
  Constant1/1 -> Div1/2
  Sum/1 -> Switch3/3
  Constant13/1 -> Switch3/1
  LogOp1/1 -> Switch3/2
  RelOp4/1 -> LogOp1/2
  RelOp3/1 -> LogOp1/1
  Constant12/1 -> RelOp4/2
  Switch3/1 -> Switch2/3
  Constant11/1 -> RelOp3/2
  Switch2/1 -> Out1/1
  RelOp2/1 -> Switch2/2
  Constant10/1 -> RelOp2/2
  In1/1 -> Div1/1, RelOp4/1, RelOp3/1, Switch2/1, RelOp2/1

== system DAS/SimToRealTime/VAPS_TimeConfiguration/RealTimeTimerAdapter_Value ==
  In1 : Inport
  Constant11 : Constant
  Constant12 : Constant  Value=-1
  Constant13 : Constant  Value=0
  LogOp1 : Logic
  RelOp3 : RelationalOperator  Operator=<=  InputSameDT=on
  RelOp4 : RelationalOperator  InputSameDT=on
  Switch3 : Switch  Threshold=1  SaturateOnIntegerOverflow=on  InputSameDT=on
  Out1 : Outport
  wires:
  In1/1 -> RelOp3/1, RelOp4/1, Switch3/3
  Switch3/1 -> Out1/1
  Constant11/1 -> RelOp3/2
  Constant12/1 -> RelOp4/2
  RelOp3/1 -> LogOp1/1
  RelOp4/1 -> LogOp1/2
  LogOp1/1 -> Switch3/2
  Constant13/1 -> Switch3/1

== system DAS/SimToRealTime/VAPS_TimeConfiguration/SysInit1 ==
  Memory_Init : UnitDelay  InitialCondition=1  SampleTime=dT
  Zero_Init : Constant  Value=0  SampleTime=dT
  y : Outport
  wires:
  Zero_Init/1 -> Memory_Init/1
  Memory_Init/1 -> y/1

== system DAS/SimToRealTime/VAPS_TimeConfiguration/VAPSRealTimeTimer ==
  TimeFactor : Inport
  Level-2 M-file S-Function : M-S-Function  FunctionName=VAPSRealTimeTimer
  TsSim : Outport
  TsRTime : Outport  Port=2
  TsRTimeEffective : Outport  Port=3
  wires:
  Level-2 M-file S-Function/3 -> TsRTimeEffective/1  "TsRTimeEffective"
  Level-2 M-file S-Function/2 -> TsRTime/1  "TsRTime"
  Level-2 M-file S-Function/1 -> TsSim/1  "TsSim"
  TimeFactor/1 -> Level-2 M-file S-Function/1

== system DAS/Umgebung/Object/Accumulator_REL ==
  MX : Inport
  MN : Inport  Port=2
  u : Inport  Port=3
  E : Inport  Port=4
  R : Inport  Port=5
  IV : Inport  Port=6
  Limit : Subsystem  mask(MSR_V200_Limit){YName=, b_maxName=, b_minName=}
      mask prompts: YName "Y OutName"; b_maxName "b_max OutName"; b_minName "b_min OutName"
      mask help:
      | Limits the input value 'u' between a maximum 'MX' and a minimum 'MN' value.
      | 'b_max' and 'b_min' indicate that the limit is exceeded.
      mask init:
      | sl_act_sg_init_blk;
      mask Help:
      | <HTML>
      | <HEAD>
      | <META HTTP-EQUIV="Content-Type" CONTENT="text/html; charset=iso-8859-1">
      | <TITLE>Help</TITLE>
      | </HEAD>
      | <BODY>
      | 
      | <B><FONT FACE="Arial"><P>Function:</P>
      | </B><P>The block limits the input signal
      |  <FONT FACE="Courier New">u</FONT> to a maximum value
      |   <FONT FACE="Courier New">MX</FONT> and a minimum value
      | 	 <FONT FACE="Courier New">MN</FONT>. First,
      | 	 <FONT FACE="Courier New">u</FONT> is checked against the maximum value,
      | 		then against the minimum value. The outputs
      | 	  <FONT FACE="Courier New">b_min</FONT> and
      | 		 <FONT FACE="Courier New">b_max</FONT> indicate a limit violation of the
      | 		  input signal <FONT FACE="Courier New">u</FONT>.</P>
      | 
      | <B><P>In-/Outputs:</P>
      | </B>
      | <P><U>Input</U></P>
      | <P>The block input <FONT FACE="Courier New">u</FONT> must be connected
      | 	 to the input signal.</P>
      | 
      | <U><P>Limit Values</P>
      | </U><P>The inputs <FONT FACE="Courier New">MN</FONT> and
      |  <FONT FACE="Courier New">MX</FONT> specify the signal value limits for
      |   <FONT FACE="Courier New">u</FONT>.</P>
      | 
      | <U><P>Output</P>
      | </U><P>The output </FONT><FONT FACE="Courier New">y</FONT>
      | <FONT FACE="Arial"> shows the input signal limited to
      |  <FONT FACE="Courier New">MN</FONT> and
      |  <FONT FACE="Courier New">MX</FONT>. A limitation is indicated by
      |   <FONT FACE="Courier New">b_min</FONT> and
      | 		 <FONT FACE="Courier New">b_max</FONT>.</P>
      | </FONT></BODY>
      | </HTML>
      mask Display: image(imread('Limiter.tif','tif'),[0.18,0.22,0.5,0.7])
  Memory_Y : UnitDelay  SampleTime=dT
  Sum_yu : Sum  SaturateOnIntegerOverflow=on  InputSameDT=on  OutDataTypeStr=Inherit: Same as first input
  Switch_E : Switch  Threshold=1  SaturateOnIntegerOverflow=on  InputSameDT=on
  Switch_R : Switch  Threshold=1  SaturateOnIntegerOverflow=on  InputSameDT=on
  y : Outport
  b_max : Outport  Port=2
  b_min : Outport  Port=3
  wires:
  R/1 -> Switch_R/2
  u/1 -> Sum_yu/1
  Sum_yu/1 -> Switch_E/1
  Switch_E/1 -> Switch_R/3
  IV/1 -> Switch_R/1
  E/1 -> Switch_E/2
  Memory_Y/1 -> Sum_yu/2, Switch_E/3
  Limit/1(y) -> y/1, Memory_Y/1
  Limit/2(b_max) -> b_max/1
  Limit/3(b_min) -> b_min/1
  MN/1 -> Limit/2(MN)
  MX/1 -> Limit/1(MX)
  Switch_R/1 -> Limit/3(u)

== system DAS/Umgebung/Vehicle/Discrete Transfer Fcn (with initial states) ==
  In1 : Inport
  Discrete State Space : DiscreteStateSpace  A=A  B=B  C=C  D=Dd  X0=X0  SampleTime=TS
  Out1 : Outport  InitialOutput=0
  wires:
  In1/1 -> Discrete State Space/1
  Discrete State Space/1 -> Out1/1
